simulink model "HelicoModel"  (R2014b)
settings: Solver=ode45  StartTime=0.0  StopTime=wSimulationTime  FixedStep=T  MaxStep=wMaxStep  RelTol=1e-3
StopFcn:
  | save(wSaveFileName,wSaveFileName)
values from neighbouring files (symbols this model uses):
  wSampleTime = 0.04    [HelicoDataDictionnary.m]
undefined symbols (not defined in the file): wComp_Tutd, wComp_Tutn, wCompDen, wCompNum, wSys_Hald, wSys_Haln, wSys_Tutd, wSys_Tutn, wSysDen, wSysNum
settings Model: Creator=Zangdaarr  LastModifiedBy=Zangdaarr

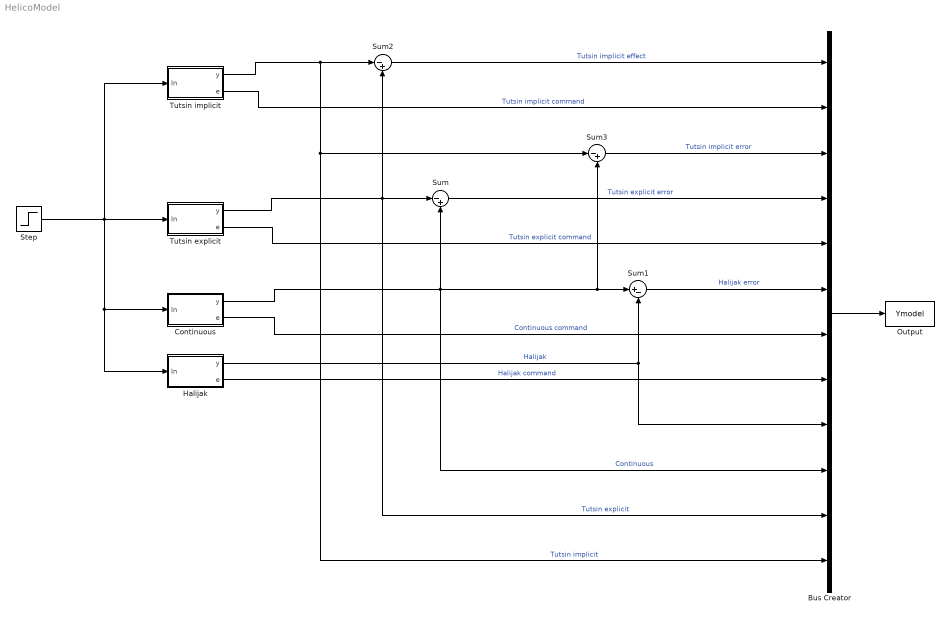
== system HelicoModel ==
  Bus Creator : BusCreator  Inputs=12
  Continuous : Subsystem  mask{S_num=wSysNum, S_den=wSysDen, C_num=wCompNum, C_den=wCompDen}
      mask prompts: S_num "System num"; S_den "System den"; C_num "Compensator num"; C_den "Compensator den"
  Halijak : Subsystem  mask{S_num=wSys_Haln, S_den=wSys_Hald, C_num=wComp_Tutn, C_den=wComp_Tutd, T=wSampleTime}
      mask prompts: S_num "System num"; S_den "System den"; C_num "Compensator num"; C_den "Compensator den"; T "Sample Time"
  Output : ToWorkspace  VariableName=Ymodel  SaveFormat=Timeseries  SampleTime=wSampleTime
  Step : Step  Time=0  After=0.1  SampleTime=0
  Sum : Sum  Inputs=|-+
  Sum1 : Sum  Inputs=|+-
  Sum2 : Sum  Inputs=|-+
  Sum3 : Sum  Inputs=|-+
  Tutsin explicit : Subsystem  mask{S_num=wSys_Tutn, S_den=wSys_Tutd, C_num=wComp_Tutn, C_den=wComp_Tutd, T=wSampleTime}
      mask prompts: S_num "System num"; S_den "System den"; C_num "Compensator num"; C_den "Compensator den"; T "Sample Time"
  Tutsin implicit : Subsystem  mask{S_num=wSys_Tutn, S_den=wSys_Tutd, C_num=wComp_Tutn, C_den=wComp_Tutd, T=wSampleTime}
      mask prompts: S_num "System num"; S_den "System den"; C_num "Compensator num"; C_den "Compensator den"; T "Sample Time"
  wires:
  Step/1 -> Tutsin implicit/1(In), Halijak/1(In), Continuous/1(In), Tutsin explicit/1(In)
  Halijak/1(y) -> Bus Creator/9, Sum1/2  "Halijak"
  Continuous/1(y) -> Sum3/2, Sum1/1, Bus Creator/10, Sum/2  "Continuous"
  Tutsin explicit/1(y) -> Sum/1, Bus Creator/11, Sum2/2  "Tutsin explicit"
  Bus Creator/1 -> Output/1
  Tutsin implicit/1(y) -> Bus Creator/12, Sum3/1, Sum2/1  "Tutsin implicit"
  Sum2/1 -> Bus Creator/1  "Tutsin implicit effect"
  Tutsin implicit/2(e) -> Bus Creator/2  "Tutsin implicit command"
  Sum3/1 -> Bus Creator/3  "Tutsin implicit error"
  Sum/1 -> Bus Creator/4  "Tutsin explicit error"
  Tutsin explicit/2(e) -> Bus Creator/5  "Tutsin explicit command"
  Sum1/1 -> Bus Creator/6  "Halijak error"
  Continuous/2(e) -> Bus Creator/7  "Continuous command"
  Halijak/2(e) -> Bus Creator/8  "Halijak command"

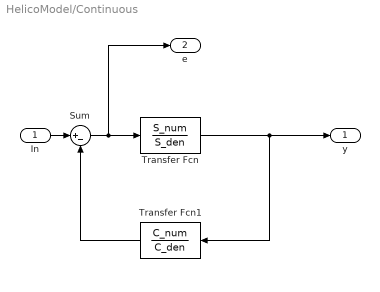
== system HelicoModel/Continuous ==
  In : Inport
  Sum : Sum  Inputs=|+-
  Transfer Fcn : TransferFcn  Numerator=S_num  Denominator=S_den
  Transfer Fcn1 : TransferFcn  Numerator=C_num  Denominator=C_den
  y : Outport
  e : Outport  Port=2
  wires:
  Transfer Fcn1/1 -> Sum/2
  In/1 -> Sum/1
  Transfer Fcn/1 -> Transfer Fcn1/1, y/1
  Sum/1 -> e/1, Transfer Fcn/1

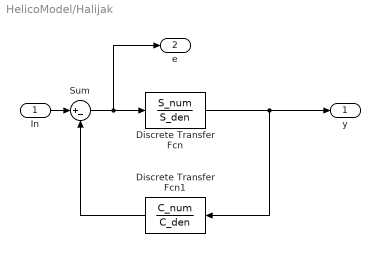
== system HelicoModel/Halijak ==
  In : Inport
  Discrete Transfer Fcn : DiscreteTransferFcn  Numerator=S_num  Denominator=S_den  SampleTime=T
  Discrete Transfer Fcn1 : DiscreteTransferFcn  Numerator=C_num  Denominator=C_den  SampleTime=T
  Sum : Sum  Inputs=|+-
  y : Outport
  e : Outport  Port=2
  wires:
  Discrete Transfer Fcn1/1 -> Sum/2
  In/1 -> Sum/1
  Discrete Transfer Fcn/1 -> y/1, Discrete Transfer Fcn1/1
  Sum/1 -> e/1, Discrete Transfer Fcn/1

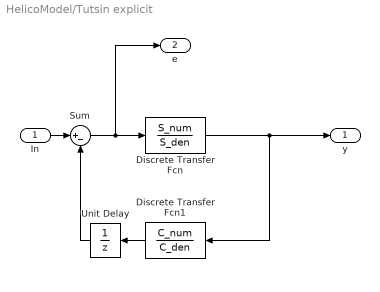
== system HelicoModel/Tutsin explicit ==
  In : Inport
  Discrete Transfer Fcn : DiscreteTransferFcn  Numerator=S_num  Denominator=S_den  SampleTime=T
  Discrete Transfer Fcn1 : DiscreteTransferFcn  Numerator=C_num  Denominator=C_den  SampleTime=T
  Sum : Sum  Inputs=|+-
  Unit Delay : UnitDelay  SampleTime=T
  y : Outport
  e : Outport  Port=2
  wires:
  Sum/1 -> e/1, Discrete Transfer Fcn/1
  Discrete Transfer Fcn/1 -> Discrete Transfer Fcn1/1, y/1
  In/1 -> Sum/1
  Discrete Transfer Fcn1/1 -> Unit Delay/1
  Unit Delay/1 -> Sum/2

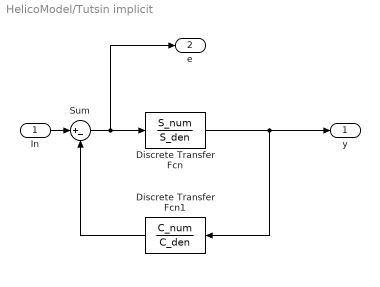
== system HelicoModel/Tutsin implicit ==
  In : Inport
  Discrete Transfer Fcn : DiscreteTransferFcn  Numerator=S_num  Denominator=S_den  SampleTime=T
  Discrete Transfer Fcn1 : DiscreteTransferFcn  Numerator=C_num  Denominator=C_den  SampleTime=T
  Sum : Sum  Inputs=|+-
  y : Outport
  e : Outport  Port=2
  wires:
  Discrete Transfer Fcn1/1 -> Sum/2
  In/1 -> Sum/1
  Discrete Transfer Fcn/1 -> y/1, Discrete Transfer Fcn1/1
  Sum/1 -> e/1, Discrete Transfer Fcn/1
